simulink model "FalconForceRendering"  (Simulink 7.0)
settings: Solver=ode1  StartTime=0.0  StopTime=inf  FixedStep=0.001  RelTol=1e-3
libraries: simulink x3, quarc_library x1
settings Model: Creator=colinlea  LastModifiedBy=colinlea  ExtModeTrigDuration=10000
settings SolverCC: PositivePriorityOrder=on
settings RTWCC: SystemTargetFile=quarc_windows.tlc  TemplateMakefile=quarc_default_tmf  Description=QuaRC Win32 Target  ProcessScript=quarc_windows_make_rtw_hook
settings STFCustomTargetCC: TargetPreCompLibLocation=C:\DOCUME~1\ALLUSE~1\APPLIC~1\QuaRC\lib\2007b\windows\release  GenFloatMathFcnCalls=ANSI_C  SystemTargetFile=quarc_windows.tlc
settings GRTTargetCC: TargetPreCompLibLocation=C:\DOCUME~1\ALLUSE~1\APPLIC~1\QuaRC\lib\2007b\windows\release  CompOptLevelCompliant=off  MatFileLogging=off  ExtMode=on  ExtModeMexFile=quarc_comm

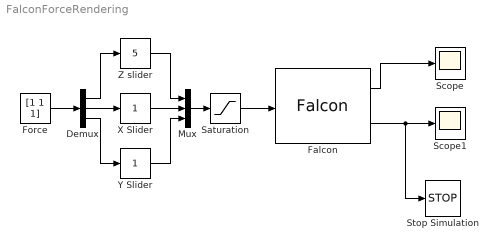
== system FalconForceRendering ==
  Demux : Demux  Outputs=3
  Falcon : quarc_library/Devices/Third-Party/Novint/Falcon  sample_time=qc_get_step_size  show_calibrate=off
  Force : Constant  Value=[1 1 1]  OutDataType=sfix(16)  OutScaling=2^0
  Mux : Mux  Inputs=3
  Saturation : Saturate  UpperLimit=10  LowerLimit=-10  OutDataType=sfix(16)  OutScaling=2^0
  Scope : Scope
      settings: TimeRange=600  YMin=-0.075  YMax=0.075
  Scope1 : Scope
      settings: TimeRange=600  YMin=0  YMax=1
  Stop Simulation : Stop
  X Slider : simulink/Math Operations/Slider Gain  SystemSampleTime=-1  low=-10  gain=1  high=10
  Y Slider : simulink/Math Operations/Slider Gain  SystemSampleTime=-1  low=-10  gain=1  high=10
  Z slider : simulink/Math Operations/Slider Gain  SystemSampleTime=-1  low=-10  gain=5  high=10
  wires:
  Falcon/1 -> Scope/1
  Falcon/2 -> Scope1/1, Stop Simulation/1
  Saturation/1 -> Falcon/1
  Z slider/1 -> Mux/1
  X Slider/1 -> Mux/2
  Y Slider/1 -> Mux/3
  Demux/1 -> Z slider/1
  Demux/2 -> X Slider/1
  Demux/3 -> Y Slider/1
  Force/1 -> Demux/1
  Mux/1 -> Saturation/1
